simulink model "animate"  (R2018a)
settings: Solver=VariableStepAuto  StartTime=0.0  StopTime=60  RelTol=1e-3
libraries: vrlib x3, dspsrcs4 x1
settings Model: OrderedModelArguments=off  Creator=Tom  LastModifiedBy=Tom

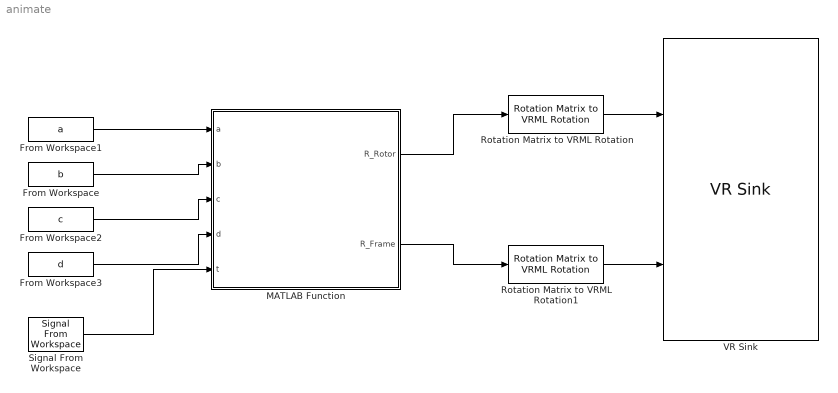
== system animate ==
  From Workspace : FromWorkspace  VariableName=b  SampleTime=0
  From Workspace1 : FromWorkspace  VariableName=a
  From Workspace2 : FromWorkspace  VariableName=c  SampleTime=0
  From Workspace3 : FromWorkspace  VariableName=d  SampleTime=0
  MATLAB Function : MATLAB Function  TreatAsAtomicUnit=on
  Rotation Matrix to VRML Rotation : vrlib/Utilities/Rotation Matrix to VRML Rotation  maxzero=1e-12
      settings: SourceProductName=Simulink 3D Animation  SourceProductBaseCode=VR
  Rotation Matrix to VRML Rotation1 : vrlib/Utilities/Rotation Matrix to VRML Rotation  maxzero=1e-12
      settings: SourceProductName=Simulink 3D Animation  SourceProductBaseCode=VR
  Signal From Workspace : dspsrcs4/Signal From Workspace  X=1:3000  Ts=0.1  nsamps=1  OutputAfterFinalValue=Holding final value  ignoreOrWarnInputAndFrameLengths=off  OutputFrames=off
  VR Sink : vrlib/VR Sink  InstantiateOnLoad=on  SampleTime=0.1  ViewEnable=on  RemoteChange=off  RemoteView=off  FieldsWritten=Rotor.rotation.4.1.1.double#Frame.rotation.4.1.1.double  WorldFileName=Simulation world.wrl  WorldDescription=Gyroscope model  AutoView=off  VideoDimensions=[500 500]  AllowVariableSize=off  FigureProperties="{'Position', 'Name', 'Viewpoint', 'CameraBound', 'CameraDirection', 'CameraPosition', 'CameraUpVector', 'ZoomFactor', 'Antialiasing', 'Headlight', 'Lighting', 'NavPanel', 'Sound', 'StatusBar', 'Stereo3D', 'Stereo3DCameraOffset', 'Stereo3DHIT', 'ToolBar', 'Textures', 'Transparency', 'Triad', 'Wireframe', 'NavZones', 'NavMode', 'NavSpeed', 'CaptureFileFormat', 'CaptureFileName', 'Record2DCompressMethod', 'Record2DCompressQuality', 'Record2D', 'Record2DFileName', 'Record2DFPS'; [2.5620000000000000e+03   8.4000000000000000e+01   9.5800000000000000e+02   9.0400000000000000e+02], 'Gyroscope model', '_untitled_2', 'on', [2.7067166547130134e-01   5.7094153312041018e-01  -7.7508877895962736e-01], [-4.8589228204951134e+01  -1.0546394456281359e+02  -1.3932617244459863e+01], [-5.5301968065827128e-02   8.1303563702122150e-01   5.7958152598363355e-01], [1.0000000000000000e+00], 'on', 'on', 'on', 'halfbar', 'on', 'on', 'off', [1.0000000149011612e-01], [0.0000000000000000e+00], 'on', 'on', 'on', 'none', 'off', 'off', 'examine', 'normal', 'tif', '%f_anim_%n.tif', 'auto', [7.5000000000000000e+01], 'off', '%f_anim_%n.avi', 'auto'; [3.0000000000000000e+01   6.0000000000000000e+01   5.0000000000000000e+02   5.0000000000000000e+02], 'Gyroscope model', '_untitled_2', 'on', [-4.9886731416417379e-01  -2.6693168704597248e-01   8.2454768043419702e-01], [8.3691543579101563e+01   9.3864891052246094e+01  -1.3975616455078125e+02], [2.6282909183113051e-01   8.5998996267187799e-01   4.3742214460500917e-01], [1.0000000000000000e+00], 'on', 'on', 'on', 'none', 'on', 'off', 'off', [1.0000000149011612e-01], [0.0000000000000000e+00], 'off', 'on', 'on', 'none', 'off', 'off', 'fly', 'normal', 'tif', '%f_anim_%n.tif', 'auto', [7.5000000000000000e+01], 'off', '***video***', 'auto'}"
      settings: SourceProductBaseCode=VR
  wires:
  From Workspace1/1 -> MATLAB Function/1(a)
  From Workspace/1 -> MATLAB Function/2(b)
  From Workspace2/1 -> MATLAB Function/3(c)
  From Workspace3/1 -> MATLAB Function/4(d)
  Rotation Matrix to VRML Rotation1/1 -> VR Sink/2
  Rotation Matrix to VRML Rotation/1 -> VR Sink/1
  Signal From Workspace/1 -> MATLAB Function/5(t)
  MATLAB Function/1(R_Rotor) -> Rotation Matrix to VRML Rotation/1
  MATLAB Function/2(R_Frame) -> Rotation Matrix to VRML Rotation1/1

== matlab function animate/MATLAB Function ==
  data: R_Rotor output size=[3 3]; R_Frame output size=[3 3]; a input; b input; c input; d input; t input
function [R_Rotor, R_Frame] = getRotations(a,b,c,d, t)
  
    a = a(t);
    b = b(t);
    c = c(t);
    d = d(t);
RFX = -[1 0 0; 0 cos(pi/2) sin(pi/2); 0 -sin(pi/2) cos(pi/2)];    
RFY = -[cos(pi/2) 0 sin(pi/2); 0 1 0; -sin(pi/2) 0 cos(pi/2)];
RFZ = [cos(3*pi/2) -sin(3*pi/2) 0; sin(3*pi/2) cos(3*pi/2) 0; 0 0 1];
    R01 = [cos(a) -sin(a) 0 ; sin(a) cos(a) 0; 0 0 1];
    R12 = [1 0 0; 0 cos(b) -sin(b); 0 sin(b) cos(b)];
    R23 = [cos(c) -sin(c) 0 ; sin(c) cos(c) 0; 0 0 1];
    R34 = [cos(d) -sin(d) 0 ; sin(d) cos(d) 0; 0 0 1];
    
    R_Frame = RFZ*RFY*R01*R12*R23*RFX;
    R_Rotor = RFZ*RFY*R01*R12*R23*R34*RFX;

end
